simulink model "example"  (R2022a)
settings: Solver=VariableStepAuto  StartTime=0.0  StopTime=10.0  RelTol=1e-3
settings Model: Creator=niranjan.bhujel  LastModifiedBy=nbhujel
settings SolverCC: AlgebraicLoopSolver=TrustRegion
settings DebuggingCC: UnconnectedInputMsg=warning  UnconnectedOutputMsg=warning  UnconnectedLineMsg=warning  SFMachineParentedDataDiag=warning

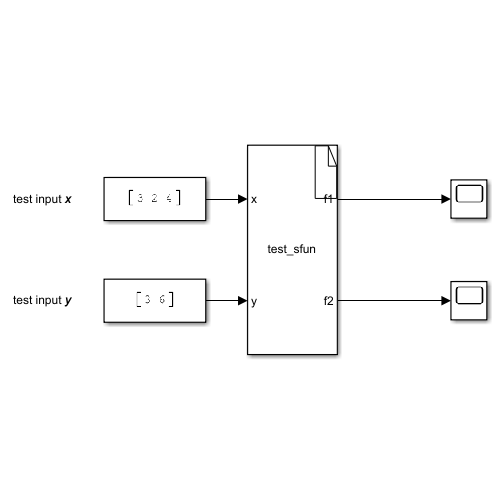
[thumbnail: Simulink's stored preview of the top-level diagram]
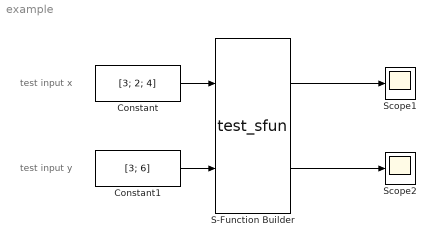
== system example ==
  note: test input x
  note: test input y
  Constant : Constant  Value=[3; 2; 4]
  Constant1 : Constant  Value=[3; 6]
  S-Function Builder : S-Function  FunctionName=test_sfun  SFunctionModules=test_sfun_wrapper test_example  SFunctionDeploymentMode=off  EnableBusSupport=off  mask(S-Function Builder){}
      mask help: Simulink:masks:SFunctionBuilder_MD
      mask init:
      | val = [[.9  0.75 0.75 1 1 .9 .9 1]',[1 1 0.75 0.75 .9 .9 1 .9]'];try , sys = get_param(gcb,'SfunBuilderFcnName');if isempty(sys), sys = get_param(gcb,'FunctionName'); end,catch, sys = get_param(gcb,'FunctionName'); end
      settings: CopyFcn=set_param(gcbh,'LinkStatus','none')  OpenFcn=sfunctionwizard(gcbh)
      mask Display:
      | plot(val(:,1),val(:,2))
      | disp(sys)
      | port_label('input',1,'x')
      | port_label('input',2,'y')
      | port_label('output',1,'f1')
      | port_label('output',2,'f2')
  Scope1 : Scope
  Scope2 : Scope
  wires:
  S-Function Builder/1 -> Scope1/1
  Constant/1 -> S-Function Builder/1
  Constant1/1 -> S-Function Builder/2
  S-Function Builder/2 -> Scope2/1
